simulink model "plant"  (R2026a)
settings: Solver=VariableStepAuto  StopTime=11
InitFcn:
  | run('plant_parameters.m');
values from neighbouring files (symbols this model uses):
  d = 0.1845    [plant_parameters.m]
  dd = d / sqrt(2)    [plant_parameters.m]
  Kd_J1 = 40    [plant_parameters.m]
  Kd_J2 = 30    [plant_parameters.m]
  Kd_J3 = 12    [plant_parameters.m]
  Ki_J1 = 800    [plant_parameters.m]
  Ki_J2 = 700    [plant_parameters.m]
  Ki_J3 = 300    [plant_parameters.m]
  Kp_J1 = 800    [plant_parameters.m]
  Kp_J2 = 600    [plant_parameters.m]
  Kp_J3 = 250    [plant_parameters.m]
  L1 = 0.074    [plant_parameters.m]
  L2 = 0.121    [plant_parameters.m]
  L3 = 0.230    (= 0.23)    [plant_parameters.m]
  N_J1 = 120    [plant_parameters.m]
  N_J2 = 120    [plant_parameters.m]
  N_J3 = 120    [plant_parameters.m]
  Sampling_Time = 0.005    [plant_parameters.m]
undefined symbols (not defined in the file or in its folder): X, Y, Z
libraries: sm_lib x121, nesl_utility x55, slpidlib x18
(part 7 of 8)

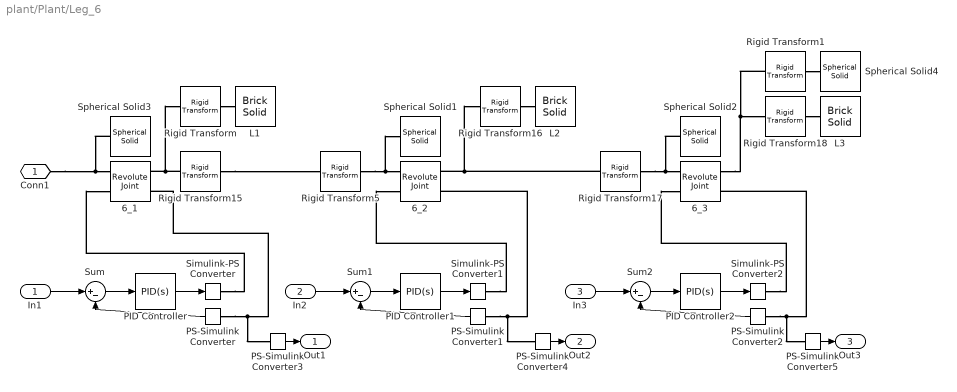
== system plant/Plant/Leg_6 ==
  In1 : Inport
  In2 : Inport  Port=2
  In3 : Inport  Port=3
  6_1 : sm_lib/Joints/Revolute Joint  JointMode=Normal  CompositeWrenchDir=FollowerOnBase  CompositeWrenchFrame=BaseFrame  SenseConstraintForce=off  SenseConstraintTorque=off  SenseTotalForce=off  SenseTotalTorque=off  PositionTargetSpecify=off  PositionTargetPriority=High  PositionTargetValue=0  PositionTargetValueUnits=deg  VelocityTargetSpecify=off  VelocityTargetPriority=High  VelocityTargetValue=0  VelocityTargetValueUnits=deg/s  EquilibriumPosition=0  EquilibriumPositionUnits=deg  SpringStiffness=0  SpringStiffnessUnits=N*m/deg  DampingCoefficient=0  DampingCoefficientUnits=N*m/(deg/s)  LowerLimitSpecify=off  LowerLimitBound=-90  LowerLimitBoundUnits=deg  LowerLimitStiffness=1e4  LowerLimitStiffnessUnits=N*m/deg  LowerLimitDamping=10  LowerLimitDampingUnits=N*m/(deg/s)  LowerLimitTransitionRegionWidth=0.1  LowerLimitTransitionRegionWidthUnits=deg  UpperLimitSpecify=off  UpperLimitBound=90  UpperLimitBoundUnits=deg  UpperLimitStiffness=1e4  UpperLimitStiffnessUnits=N*m/deg  UpperLimitDamping=10  UpperLimitDampingUnits=N*m/(deg/s)  UpperLimitTransitionRegionWidth=0.1  UpperLimitTransitionRegionWidthUnits=deg  TorqueActuationMode=InputTorque  MotionActuationMode=ComputedMotion  SensePosition=on  SenseVelocity=off  SenseAcceleration=off  SenseTorqueForce=off  SenseLowerLimitTorqueForce=off  SenseUpperLimitTorqueForce=off
  6_2 : sm_lib/Joints/Revolute Joint  JointMode=Normal  CompositeWrenchDir=FollowerOnBase  CompositeWrenchFrame=BaseFrame  SenseConstraintForce=off  SenseConstraintTorque=off  SenseTotalForce=off  SenseTotalTorque=off  PositionTargetSpecify=off  PositionTargetPriority=High  PositionTargetValue=0  PositionTargetValueUnits=deg  VelocityTargetSpecify=off  VelocityTargetPriority=High  VelocityTargetValue=0  VelocityTargetValueUnits=deg/s  EquilibriumPosition=0  EquilibriumPositionUnits=deg  SpringStiffness=0  SpringStiffnessUnits=N*m/deg  DampingCoefficient=0  DampingCoefficientUnits=N*m/(deg/s)  LowerLimitSpecify=off  LowerLimitBound=-90  LowerLimitBoundUnits=deg  LowerLimitStiffness=1e4  LowerLimitStiffnessUnits=N*m/deg  LowerLimitDamping=10  LowerLimitDampingUnits=N*m/(deg/s)  LowerLimitTransitionRegionWidth=0.1  LowerLimitTransitionRegionWidthUnits=deg  UpperLimitSpecify=off  UpperLimitBound=90  UpperLimitBoundUnits=deg  UpperLimitStiffness=1e4  UpperLimitStiffnessUnits=N*m/deg  UpperLimitDamping=10  UpperLimitDampingUnits=N*m/(deg/s)  UpperLimitTransitionRegionWidth=0.1  UpperLimitTransitionRegionWidthUnits=deg  TorqueActuationMode=InputTorque  MotionActuationMode=ComputedMotion  SensePosition=on  SenseVelocity=off  SenseAcceleration=off  SenseTorqueForce=off  SenseLowerLimitTorqueForce=off  SenseUpperLimitTorqueForce=off
  6_3 : sm_lib/Joints/Revolute Joint  JointMode=Normal  CompositeWrenchDir=FollowerOnBase  CompositeWrenchFrame=BaseFrame  SenseConstraintForce=off  SenseConstraintTorque=off  SenseTotalForce=off  SenseTotalTorque=off  PositionTargetSpecify=off  PositionTargetPriority=High  PositionTargetValue=0  PositionTargetValueUnits=deg  VelocityTargetSpecify=off  VelocityTargetPriority=High  VelocityTargetValue=0  VelocityTargetValueUnits=deg/s  EquilibriumPosition=0  EquilibriumPositionUnits=deg  SpringStiffness=0  SpringStiffnessUnits=N*m/deg  DampingCoefficient=0  DampingCoefficientUnits=N*m/(deg/s)  LowerLimitSpecify=off  LowerLimitBound=-90  LowerLimitBoundUnits=deg  LowerLimitStiffness=1e4  LowerLimitStiffnessUnits=N*m/deg  LowerLimitDamping=10  LowerLimitDampingUnits=N*m/(deg/s)  LowerLimitTransitionRegionWidth=0.1  LowerLimitTransitionRegionWidthUnits=deg  UpperLimitSpecify=off  UpperLimitBound=90  UpperLimitBoundUnits=deg  UpperLimitStiffness=1e4  UpperLimitStiffnessUnits=N*m/deg  UpperLimitDamping=10  UpperLimitDampingUnits=N*m/(deg/s)  UpperLimitTransitionRegionWidth=0.1  UpperLimitTransitionRegionWidthUnits=deg  TorqueActuationMode=InputTorque  MotionActuationMode=ComputedMotion  SensePosition=on  SenseVelocity=off  SenseAcceleration=off  SenseTorqueForce=off  SenseLowerLimitTorqueForce=off  SenseUpperLimitTorqueForce=off
  L1 : sm_lib/Body Elements/Brick Solid  BrickDimensions=[L1 0.05 0.05]  BrickDimensionsUnits=m  ExportEntireGeometry=off  InertiaType=CalculateFromGeometry  BasedOnType=Density  Density=1000  DensityUnits=kg/m^3  Mass=1  MassUnits=kg  CenterOfMass=[0 0 0]  CenterOfMassUnits=m  MomentsOfInertia=[1 1 1]  MomentsOfInertiaUnits=kg*m^2  ProductsOfInertia=[0 0 0]  ProductsOfInertiaUnits=kg*m^2  GraphicType=FromGeometry  MarkerShape=Sphere  MarkerSize=10  GraphicVisPropType=SimpleVisualProperties  GraphicDiffuseColor=[0.5 0.5 0.5]  GraphicOpacity=1  GraphicSpecularColor=[0.5 0.5 0.5 1.0]  GraphicAmbientColor=[0.15 0.15 0.15 1.0]  GraphicEmissiveColor=[0.0 0.0 0.0 1.0]  GraphicShininess=75  DoExposeReferenceFrame=on  SerializedFrames=<Frames/>
  L2 : sm_lib/Body Elements/Brick Solid  BrickDimensions=[L2 0.05 0.05]  BrickDimensionsUnits=m  ExportEntireGeometry=off  InertiaType=CalculateFromGeometry  BasedOnType=Density  Density=1000  DensityUnits=kg/m^3  Mass=1  MassUnits=kg  CenterOfMass=[0 0 0]  CenterOfMassUnits=m  MomentsOfInertia=[1 1 1]  MomentsOfInertiaUnits=kg*m^2  ProductsOfInertia=[0 0 0]  ProductsOfInertiaUnits=kg*m^2  GraphicType=FromGeometry  MarkerShape=Sphere  MarkerSize=10  GraphicVisPropType=SimpleVisualProperties  GraphicDiffuseColor=[0.5 0.5 0.5]  GraphicOpacity=1  GraphicSpecularColor=[0.5 0.5 0.5 1.0]  GraphicAmbientColor=[0.15 0.15 0.15 1.0]  GraphicEmissiveColor=[0.0 0.0 0.0 1.0]  GraphicShininess=75  DoExposeReferenceFrame=on  SerializedFrames=<Frames/>
  L3 : sm_lib/Body Elements/Brick Solid  BrickDimensions=[L3 0.05 0.05]  BrickDimensionsUnits=m  ExportEntireGeometry=off  InertiaType=CalculateFromGeometry  BasedOnType=Density  Density=1000  DensityUnits=kg/m^3  Mass=1  MassUnits=kg  CenterOfMass=[0 0 0]  CenterOfMassUnits=m  MomentsOfInertia=[1 1 1]  MomentsOfInertiaUnits=kg*m^2  ProductsOfInertia=[0 0 0]  ProductsOfInertiaUnits=kg*m^2  GraphicType=FromGeometry  MarkerShape=Sphere  MarkerSize=10  GraphicVisPropType=SimpleVisualProperties  GraphicDiffuseColor=[0.5 0.5 0.5]  GraphicOpacity=1  GraphicSpecularColor=[0.5 0.5 0.5 1.0]  GraphicAmbientColor=[0.15 0.15 0.15 1.0]  GraphicEmissiveColor=[0.0 0.0 0.0 1.0]  GraphicShininess=75  DoExposeReferenceFrame=on  SerializedFrames=<Frames/>
  PID Controller : slpidlib/PID Controller  Controller=PID  Form=Parallel  TimeDomain=Continuous-time  UseExternalTs=off  SampleTime=-1  IntegratorMethod=Forward Euler  FilterMethod=Forward Euler  ControllerParametersSource=internal  P=Kp_J1  I=Ki_J1  UseKiTs=off  D=Kd_J1  UseExternalDerivativeSource=off  N=N_J1  UseFilter=on  TunerSelectOption=Transfer Function Based (PID Tuner App)  InitialConditionSource=internal  InitialConditionForIntegrator=0  InitialConditionForFilter=0  DifferentiatorICPrevScaledInput=0  ExternalReset=none  TrackingMode=off  Kt=1  LimitOutput=off  SatLimitsSource=internal  UpperSaturationLimit=inf  LowerSaturationLimit=-inf  LinearizeAsGain=on  AntiWindupMode=none  Kb=1  LimitIntegrator=off  UpperIntegratorSaturationLimit=inf  LowerIntegratorSaturationLimit=-inf  POutMin=[]  POutMax=[]  IOutMin=[]  IOutMax=[]  DOutMin=[]  DOutMax=[]  NOutMin=[]  NOutMax=[]  SumOutMin=[]  SumOutMax=[]  SaturationOutMin=[]  SaturationOutMax=[]  PParamMin=[]  PParamMax=[]  IParamMin=[]  IParamMax=[]  DParamMin=[]  DParamMax=[]  NParamMin=[]  NParamMax=[]  KbParamMin=[]  KbParamMax=[]  KtParamMin=[]  KtParamMax=[]  KbOutMin=[]  KbOutMax=[]  KtOutMin=[]  KtOutMax=[]  IntegratorOutMin=[]  IntegratorOutMax=[]  FilterOutMin=[]  FilterOutMax=[]  SumI1OutMin=[]  SumI1OutMax=[]  SumI2OutMin=[]  SumI2OutMax=[]  SumI3OutMin=[]  SumI3OutMax=[]  SumI4OutMin=[]  SumI4OutMax=[]  SumDOutMin=[]  SumDOutMax=[]  DifferentiatorOutMin=[]  DifferentiatorOutMax=[]  FilterDiffOutCoefMin=[]  FilterDiffOutCoefMax=[]  ReciprocalOutMin=[]  ReciprocalOutMax=[]  SumDenOutMin=[]  SumDenOutMax=[]  SumNumOutMin=[]  SumNumOutMax=[]  DivideOutMin=[]  DivideOutMax=[]  UdiffTsProdOutMin=[]  UdiffTsProdOutMax=[]  NTsProdOutMin=[]  NTsProdOutMax=[]  UintegralTsProdOutMin=[]  UintegralTsProdOutMax=[]  UngainTsProdOutMin=[]  UngainTsProdOutMax=[]  ClampingZeroOutDataTypeStr=Inherit: Inherit via back propagation  ClampingZeroOutMin=[]  ClampingZeroOutMax=[]  FilterDenConstantOutDataTypeStr=Inherit: Inherit via back propagation  FilterDenConstantOutMin=[]  FilterDenConstantOutMax=[]  PCopyOutDataTypeStr=Inherit: Inherit via back propagation  PCopyOutMin=[]  PCopyOutMax=[]  NCopyOutDataTypeStr=Inherit: Inherit via back propagation  NCopyOutMin=[]  NCopyOutMax=[]  IntegratorContinuousStateAttributes=''  IntegratorStateMustResolveToSignalObject=off  IntegratorRTWStateStorageClass=Auto  FilterContinuousStateAttributes=''  FilterStateMustResolveToSignalObject=off  FilterRTWStateStorageClass=Auto  ParallelPVariant=InternalParameters  IdealPVariant=Disabled  IVariant=InternalParameters  DVariant=InternalParameters  IntegratorVariant=Continuous  SatVariant=Disabled  AWVariant=Passthrough  PCopyVariant=Disabled  TRVariant=Disabled  FdbkBlocksVariant=Forward  IdealPFdbkVariant=Disabled  SatFdbkVariant=Disabled  DerivativeFilterVariant=ContFilter  NVariant=InternalParameters  NCopyVariant=Disabled  FilterICVariant=InternalICsFilter  IntegratorICVariant=InternalICs  ExternalResetVariant=Disabled  TRSumVariant=Passthrough  SumFdbkVariant=Disabled  SumVariant=Sum_PID  TsampFilterVariant=InternalTs  TsampNgainVariant=Passthrough  TsampIntegralVariant=Disabled_SignalSpec  ExternalSaturationOutDataTypeStr=Inherit: Same as second input  DerivativeSourceVariant=ErrorSignal  PreIntVariant=InternalPreInt
  PID Controller1 : slpidlib/PID Controller  Controller=PID  Form=Parallel  TimeDomain=Continuous-time  UseExternalTs=off  SampleTime=-1  IntegratorMethod=Forward Euler  FilterMethod=Forward Euler  ControllerParametersSource=internal  P=Kp_J2  I=Ki_J2  UseKiTs=off  D=Kd_J2  UseExternalDerivativeSource=off  N=N_J2  UseFilter=on  TunerSelectOption=Transfer Function Based (PID Tuner App)  InitialConditionSource=internal  InitialConditionForIntegrator=0  InitialConditionForFilter=0  DifferentiatorICPrevScaledInput=0  ExternalReset=none  TrackingMode=off  Kt=1  LimitOutput=off  SatLimitsSource=internal  UpperSaturationLimit=inf  LowerSaturationLimit=-inf  LinearizeAsGain=on  AntiWindupMode=none  Kb=1  LimitIntegrator=off  UpperIntegratorSaturationLimit=inf  LowerIntegratorSaturationLimit=-inf  POutMin=[]  POutMax=[]  IOutMin=[]  IOutMax=[]  DOutMin=[]  DOutMax=[]  NOutMin=[]  NOutMax=[]  SumOutMin=[]  SumOutMax=[]  SaturationOutMin=[]  SaturationOutMax=[]  PParamMin=[]  PParamMax=[]  IParamMin=[]  IParamMax=[]  DParamMin=[]  DParamMax=[]  NParamMin=[]  NParamMax=[]  KbParamMin=[]  KbParamMax=[]  KtParamMin=[]  KtParamMax=[]  KbOutMin=[]  KbOutMax=[]  KtOutMin=[]  KtOutMax=[]  IntegratorOutMin=[]  IntegratorOutMax=[]  FilterOutMin=[]  FilterOutMax=[]  SumI1OutMin=[]  SumI1OutMax=[]  SumI2OutMin=[]  SumI2OutMax=[]  SumI3OutMin=[]  SumI3OutMax=[]  SumI4OutMin=[]  SumI4OutMax=[]  SumDOutMin=[]  SumDOutMax=[]  DifferentiatorOutMin=[]  DifferentiatorOutMax=[]  FilterDiffOutCoefMin=[]  FilterDiffOutCoefMax=[]  ReciprocalOutMin=[]  ReciprocalOutMax=[]  SumDenOutMin=[]  SumDenOutMax=[]  SumNumOutMin=[]  SumNumOutMax=[]  DivideOutMin=[]  DivideOutMax=[]  UdiffTsProdOutMin=[]  UdiffTsProdOutMax=[]  NTsProdOutMin=[]  NTsProdOutMax=[]  UintegralTsProdOutMin=[]  UintegralTsProdOutMax=[]  UngainTsProdOutMin=[]  UngainTsProdOutMax=[]  ClampingZeroOutDataTypeStr=Inherit: Inherit via back propagation  ClampingZeroOutMin=[]  ClampingZeroOutMax=[]  FilterDenConstantOutDataTypeStr=Inherit: Inherit via back propagation  FilterDenConstantOutMin=[]  FilterDenConstantOutMax=[]  PCopyOutDataTypeStr=Inherit: Inherit via back propagation  PCopyOutMin=[]  PCopyOutMax=[]  NCopyOutDataTypeStr=Inherit: Inherit via back propagation  NCopyOutMin=[]  NCopyOutMax=[]  IntegratorContinuousStateAttributes=''  IntegratorStateMustResolveToSignalObject=off  IntegratorRTWStateStorageClass=Auto  FilterContinuousStateAttributes=''  FilterStateMustResolveToSignalObject=off  FilterRTWStateStorageClass=Auto  ParallelPVariant=InternalParameters  IdealPVariant=Disabled  IVariant=InternalParameters  DVariant=InternalParameters  IntegratorVariant=Continuous  SatVariant=Disabled  AWVariant=Passthrough  PCopyVariant=Disabled  TRVariant=Disabled  FdbkBlocksVariant=Forward  IdealPFdbkVariant=Disabled  SatFdbkVariant=Disabled  DerivativeFilterVariant=ContFilter  NVariant=InternalParameters  NCopyVariant=Disabled  FilterICVariant=InternalICsFilter  IntegratorICVariant=InternalICs  ExternalResetVariant=Disabled  TRSumVariant=Passthrough  SumFdbkVariant=Disabled  SumVariant=Sum_PID  TsampFilterVariant=InternalTs  TsampNgainVariant=Passthrough  TsampIntegralVariant=Disabled_SignalSpec  ExternalSaturationOutDataTypeStr=Inherit: Same as second input  DerivativeSourceVariant=ErrorSignal  PreIntVariant=InternalPreInt
  PID Controller2 : slpidlib/PID Controller  Controller=PID  Form=Parallel  TimeDomain=Continuous-time  UseExternalTs=off  SampleTime=-1  IntegratorMethod=Forward Euler  FilterMethod=Forward Euler  ControllerParametersSource=internal  P=Kp_J3  I=Ki_J3  UseKiTs=off  D=Kd_J3  UseExternalDerivativeSource=off  N=N_J3  UseFilter=on  TunerSelectOption=Transfer Function Based (PID Tuner App)  InitialConditionSource=internal  InitialConditionForIntegrator=0  InitialConditionForFilter=0  DifferentiatorICPrevScaledInput=0  ExternalReset=none  TrackingMode=off  Kt=1  LimitOutput=off  SatLimitsSource=internal  UpperSaturationLimit=inf  LowerSaturationLimit=-inf  LinearizeAsGain=on  AntiWindupMode=none  Kb=1  LimitIntegrator=off  UpperIntegratorSaturationLimit=inf  LowerIntegratorSaturationLimit=-inf  POutMin=[]  POutMax=[]  IOutMin=[]  IOutMax=[]  DOutMin=[]  DOutMax=[]  NOutMin=[]  NOutMax=[]  SumOutMin=[]  SumOutMax=[]  SaturationOutMin=[]  SaturationOutMax=[]  PParamMin=[]  PParamMax=[]  IParamMin=[]  IParamMax=[]  DParamMin=[]  DParamMax=[]  NParamMin=[]  NParamMax=[]  KbParamMin=[]  KbParamMax=[]  KtParamMin=[]  KtParamMax=[]  KbOutMin=[]  KbOutMax=[]  KtOutMin=[]  KtOutMax=[]  IntegratorOutMin=[]  IntegratorOutMax=[]  FilterOutMin=[]  FilterOutMax=[]  SumI1OutMin=[]  SumI1OutMax=[]  SumI2OutMin=[]  SumI2OutMax=[]  SumI3OutMin=[]  SumI3OutMax=[]  SumI4OutMin=[]  SumI4OutMax=[]  SumDOutMin=[]  SumDOutMax=[]  DifferentiatorOutMin=[]  DifferentiatorOutMax=[]  FilterDiffOutCoefMin=[]  FilterDiffOutCoefMax=[]  ReciprocalOutMin=[]  ReciprocalOutMax=[]  SumDenOutMin=[]  SumDenOutMax=[]  SumNumOutMin=[]  SumNumOutMax=[]  DivideOutMin=[]  DivideOutMax=[]  UdiffTsProdOutMin=[]  UdiffTsProdOutMax=[]  NTsProdOutMin=[]  NTsProdOutMax=[]  UintegralTsProdOutMin=[]  UintegralTsProdOutMax=[]  UngainTsProdOutMin=[]  UngainTsProdOutMax=[]  ClampingZeroOutDataTypeStr=Inherit: Inherit via back propagation  ClampingZeroOutMin=[]  ClampingZeroOutMax=[]  FilterDenConstantOutDataTypeStr=Inherit: Inherit via back propagation  FilterDenConstantOutMin=[]  FilterDenConstantOutMax=[]  PCopyOutDataTypeStr=Inherit: Inherit via back propagation  PCopyOutMin=[]  PCopyOutMax=[]  NCopyOutDataTypeStr=Inherit: Inherit via back propagation  NCopyOutMin=[]  NCopyOutMax=[]  IntegratorContinuousStateAttributes=''  IntegratorStateMustResolveToSignalObject=off  IntegratorRTWStateStorageClass=Auto  FilterContinuousStateAttributes=''  FilterStateMustResolveToSignalObject=off  FilterRTWStateStorageClass=Auto  ParallelPVariant=InternalParameters  IdealPVariant=Disabled  IVariant=InternalParameters  DVariant=InternalParameters  IntegratorVariant=Continuous  SatVariant=Disabled  AWVariant=Passthrough  PCopyVariant=Disabled  TRVariant=Disabled  FdbkBlocksVariant=Forward  IdealPFdbkVariant=Disabled  SatFdbkVariant=Disabled  DerivativeFilterVariant=ContFilter  NVariant=InternalParameters  NCopyVariant=Disabled  FilterICVariant=InternalICsFilter  IntegratorICVariant=InternalICs  ExternalResetVariant=Disabled  TRSumVariant=Passthrough  SumFdbkVariant=Disabled  SumVariant=Sum_PID  TsampFilterVariant=InternalTs  TsampNgainVariant=Passthrough  TsampIntegralVariant=Disabled_SignalSpec  ExternalSaturationOutDataTypeStr=Inherit: Same as second input  DerivativeSourceVariant=ErrorSignal  PreIntVariant=InternalPreInt
  PS-Simulink Converter{,1..5} (6 alike) : nesl_utility/PS-Simulink Converter  PhysicalDomain=network_engine_domain  SubClassName=ps_output  LeftPortType=input  RightPortType=output  PseudoPeriodic=off  Frequencies=[]  VectorFormat=inherit  Unit=inherit  AffineConversion=off
  Rigid Transform : sm_lib/Frames and Transforms/Rigid Transform  RotationMethod=None  FollAlignAxisA=+X  BaseAlignAxisA=+Y  FollAlignAxisB=+Y  BaseAlignAxisB=+Z  RotationStandardAxis=+Z  RotationAngle=0  RotationAngleUnits=deg  RotationArbitraryAxis=[0 0 1]  RotationSequenceAxes=FollowerAxes  RotationSequence=XYX  RotationSequenceAngles=[0 0 0]  RotationSequenceAnglesUnits=deg  RotationMatrix=[1 0 0;0 1 0;0 0 1]  Quaternion=[1 0 0 0]  TranslationMethod=Cartesian  TranslationCartesianOffset=[L1/2 0 0]  TranslationCartesianOffsetUnits=m  TranslationStandardAxis=+Z  TranslationStandardOffset=0  TranslationStandardOffsetUnits=m  TranslationROffset=0  TranslationROffsetUnits=m  TranslationThetaOffset=0  TranslationThetaOffsetUnits=deg  TranslationZOffset=0  TranslationZOffsetUnits=m
  Rigid Transform1 : sm_lib/Frames and Transforms/Rigid Transform  RotationMethod=None  FollAlignAxisA=+X  BaseAlignAxisA=+Y  FollAlignAxisB=+Y  BaseAlignAxisB=+Z  RotationStandardAxis=+Z  RotationAngle=0  RotationAngleUnits=deg  RotationArbitraryAxis=[0 0 1]  RotationSequenceAxes=FollowerAxes  RotationSequence=XYX  RotationSequenceAngles=[0 0 0]  RotationSequenceAnglesUnits=deg  RotationMatrix=[1 0 0;0 1 0;0 0 1]  Quaternion=[1 0 0 0]  TranslationMethod=Cartesian  TranslationCartesianOffset=[L3 0 0]  TranslationCartesianOffsetUnits=m  TranslationStandardAxis=+Z  TranslationStandardOffset=0  TranslationStandardOffsetUnits=m  TranslationROffset=0  TranslationROffsetUnits=m  TranslationThetaOffset=0  TranslationThetaOffsetUnits=deg  TranslationZOffset=0  TranslationZOffsetUnits=m
  Rigid Transform15 : sm_lib/Frames and Transforms/Rigid Transform  RotationMethod=None  FollAlignAxisA=+X  BaseAlignAxisA=+Y  FollAlignAxisB=+Y  BaseAlignAxisB=+Z  RotationStandardAxis=+Z  RotationAngle=0  RotationAngleUnits=deg  RotationArbitraryAxis=[0 0 1]  RotationSequenceAxes=FollowerAxes  RotationSequence=XYX  RotationSequenceAngles=[0 0 0]  RotationSequenceAnglesUnits=deg  RotationMatrix=[1 0 0;0 1 0;0 0 1]  Quaternion=[1 0 0 0]  TranslationMethod=Cartesian  TranslationCartesianOffset=[L1 0 0]  TranslationCartesianOffsetUnits=m  TranslationStandardAxis=+Z  TranslationStandardOffset=0  TranslationStandardOffsetUnits=m  TranslationROffset=0  TranslationROffsetUnits=m  TranslationThetaOffset=0  TranslationThetaOffsetUnits=deg  TranslationZOffset=0  TranslationZOffsetUnits=m
  Rigid Transform16 : sm_lib/Frames and Transforms/Rigid Transform  RotationMethod=None  FollAlignAxisA=+X  BaseAlignAxisA=+Y  FollAlignAxisB=+Y  BaseAlignAxisB=+Z  RotationStandardAxis=+Z  RotationAngle=0  RotationAngleUnits=deg  RotationArbitraryAxis=[0 0 1]  RotationSequenceAxes=FollowerAxes  RotationSequence=XYX  RotationSequenceAngles=[0 0 0]  RotationSequenceAnglesUnits=deg  RotationMatrix=[1 0 0;0 1 0;0 0 1]  Quaternion=[1 0 0 0]  TranslationMethod=Cartesian  TranslationCartesianOffset=[L2/2 0 0]  TranslationCartesianOffsetUnits=m  TranslationStandardAxis=+Z  TranslationStandardOffset=0  TranslationStandardOffsetUnits=m  TranslationROffset=0  TranslationROffsetUnits=m  TranslationThetaOffset=0  TranslationThetaOffsetUnits=deg  TranslationZOffset=0  TranslationZOffsetUnits=m
  Rigid Transform17 : sm_lib/Frames and Transforms/Rigid Transform  RotationMethod=None  FollAlignAxisA=+X  BaseAlignAxisA=+Y  FollAlignAxisB=+Y  BaseAlignAxisB=+Z  RotationStandardAxis=+Z  RotationAngle=0  RotationAngleUnits=deg  RotationArbitraryAxis=[0 0 1]  RotationSequenceAxes=FollowerAxes  RotationSequence=XYX  RotationSequenceAngles=[0 0 0]  RotationSequenceAnglesUnits=deg  RotationMatrix=[1 0 0;0 1 0;0 0 1]  Quaternion=[1 0 0 0]  TranslationMethod=Cartesian  TranslationCartesianOffset=[L2 0 0]  TranslationCartesianOffsetUnits=m  TranslationStandardAxis=+Z  TranslationStandardOffset=0  TranslationStandardOffsetUnits=m  TranslationROffset=0  TranslationROffsetUnits=m  TranslationThetaOffset=0  TranslationThetaOffsetUnits=deg  TranslationZOffset=0  TranslationZOffsetUnits=m
  Rigid Transform18 : sm_lib/Frames and Transforms/Rigid Transform  RotationMethod=None  FollAlignAxisA=+X  BaseAlignAxisA=+Y  FollAlignAxisB=+Y  BaseAlignAxisB=+Z  RotationStandardAxis=+Z  RotationAngle=0  RotationAngleUnits=deg  RotationArbitraryAxis=[0 0 1]  RotationSequenceAxes=FollowerAxes  RotationSequence=XYX  RotationSequenceAngles=[0 0 0]  RotationSequenceAnglesUnits=deg  RotationMatrix=[1 0 0;0 1 0;0 0 1]  Quaternion=[1 0 0 0]  TranslationMethod=Cartesian  TranslationCartesianOffset=[L3/2 0 0]  TranslationCartesianOffsetUnits=m  TranslationStandardAxis=+Z  TranslationStandardOffset=0  TranslationStandardOffsetUnits=m  TranslationROffset=0  TranslationROffsetUnits=m  TranslationThetaOffset=0  TranslationThetaOffsetUnits=deg  TranslationZOffset=0  TranslationZOffsetUnits=m
  Rigid Transform5 : sm_lib/Frames and Transforms/Rigid Transform  RotationMethod=StandardAxis  FollAlignAxisA=+X  BaseAlignAxisA=+Y  FollAlignAxisB=+Y  BaseAlignAxisB=+Z  RotationStandardAxis=-X  RotationAngle=90  RotationAngleUnits=deg  RotationArbitraryAxis=[0 0 1]  RotationSequenceAxes=FollowerAxes  RotationSequence=XYX  RotationSequenceAngles=[0 0 0]  RotationSequenceAnglesUnits=deg  RotationMatrix=[1 0 0;0 1 0;0 0 1]  Quaternion=[1 0 0 0]  TranslationMethod=None  TranslationCartesianOffset=[L1 0 0]  TranslationCartesianOffsetUnits=m  TranslationStandardAxis=+Z  TranslationStandardOffset=0  TranslationStandardOffsetUnits=m  TranslationROffset=0  TranslationROffsetUnits=m  TranslationThetaOffset=0  TranslationThetaOffsetUnits=deg  TranslationZOffset=0  TranslationZOffsetUnits=m
  Simulink-PS Converter : nesl_utility/Simulink-PS Converter  PhysicalDomain=network_engine_domain  SubClassName=ps_input  LeftPortType=input  RightPortType=output  PseudoPeriodic=off  Frequencies=[]  NoiseDistribution=none  NoiseParameters=[]  Unit=1  AffineConversion=off  FilteringAndDerivatives=provide  SimscapeFilterOrder=1  InputFilterTimeConstant=0.001  UdotUserProvided=0
  Simulink-PS Converter1 : nesl_utility/Simulink-PS Converter  PhysicalDomain=network_engine_domain  SubClassName=ps_input  LeftPortType=input  RightPortType=output  PseudoPeriodic=off  Frequencies=[]  NoiseDistribution=none  NoiseParameters=[]  Unit=1  AffineConversion=off  FilteringAndDerivatives=provide  SimscapeFilterOrder=1  InputFilterTimeConstant=0.001  UdotUserProvided=0
  Simulink-PS Converter2 : nesl_utility/Simulink-PS Converter  PhysicalDomain=network_engine_domain  SubClassName=ps_input  LeftPortType=input  RightPortType=output  PseudoPeriodic=off  Frequencies=[]  NoiseDistribution=none  NoiseParameters=[]  Unit=1  AffineConversion=off  FilteringAndDerivatives=provide  SimscapeFilterOrder=1  InputFilterTimeConstant=0.001  UdotUserProvided=0
  Spherical Solid{1..4} (4 alike) : sm_lib/Body Elements/Spherical Solid  SphereRadius=0.044  SphereRadiusUnits=m  ExportEntireGeometry=off  InertiaType=CalculateFromGeometry  BasedOnType=Density  Density=1000  DensityUnits=kg/m^3  Mass=1  MassUnits=kg  CenterOfMass=[0 0 0]  CenterOfMassUnits=m  MomentsOfInertia=[1 1 1]  MomentsOfInertiaUnits=kg*m^2  ProductsOfInertia=[0 0 0]  ProductsOfInertiaUnits=kg*m^2  GraphicType=FromGeometry  MarkerShape=Sphere  MarkerSize=10  GraphicVisPropType=SimpleVisualProperties  GraphicDiffuseColor=[0 0.3333 1]  GraphicOpacity=1  GraphicSpecularColor=[0.5 0.5 0.5 1.0]  GraphicAmbientColor=[0.15 0.15 0.15 1.0]  GraphicEmissiveColor=[0.0 0.0 0.0 1.0]  GraphicShininess=75  DoExposeReferenceFrame=on  SerializedFrames=<Frames/>
  Sum : Sum  Inputs=|+-
  Sum1 : Sum  Inputs=|+-
  Sum2 : Sum  Inputs=|+-
  Conn1 : PMIOPort  Side=Left
  Out1 : Outport
  Out2 : Outport  Port=2
  Out3 : Outport  Port=3
  wires:
  PID Controller/1 -> Simulink-PS Converter/1
  Sum1/1 -> PID Controller1/1
  In2/1 -> Sum1/1
  Sum/1 -> PID Controller/1
  In3/1 -> Sum2/1
  PID Controller2/1 -> Simulink-PS Converter2/1
  In1/1 -> Sum/1
  PS-Simulink Converter/1 -> Sum/2
  PS-Simulink Converter1/1 -> Sum1/2
  PS-Simulink Converter2/1 -> Sum2/2
  Sum2/1 -> PID Controller2/1
  PID Controller1/1 -> Simulink-PS Converter1/1
  PS-Simulink Converter3/1 -> Out1/1
  PS-Simulink Converter4/1 -> Out2/1
  PS-Simulink Converter5/1 -> Out3/1
  connections:
  Rigid Transform/RConn1 -- L1/RConn1
  Rigid Transform16/RConn1 -- L2/RConn1
  Rigid Transform15/RConn1 -- Rigid Transform5/LConn1
  6_3/RConn2 -- PS-Simulink Converter2/LConn1 -- PS-Simulink Converter5/LConn1
  Rigid Transform17/LConn1 -- Rigid Transform16/LConn1 -- 6_2/RConn1
  Rigid Transform17/RConn1 -- Spherical Solid2/RConn1 -- 6_3/LConn1
  Rigid Transform5/RConn1 -- Spherical Solid1/RConn1 -- 6_2/LConn1
  Simulink-PS Converter/RConn1 -- 6_1/LConn2
  Simulink-PS Converter1/RConn1 -- 6_2/LConn2
  6_3/RConn1 -- Rigid Transform1/LConn1 -- Rigid Transform18/LConn1
  Rigid Transform15/LConn1 -- Rigid Transform/LConn1 -- 6_1/RConn1
  Rigid Transform18/RConn1 -- L3/RConn1
  6_2/RConn2 -- PS-Simulink Converter1/LConn1 -- PS-Simulink Converter4/LConn1
  PS-Simulink Converter/LConn1 -- 6_1/RConn2 -- PS-Simulink Converter3/LConn1
  Conn1/RConn1 -- Spherical Solid3/RConn1 -- 6_1/LConn1
  Simulink-PS Converter2/RConn1 -- 6_3/LConn2
  Rigid Transform1/RConn1 -- Spherical Solid4/RConn1

== matlab function plant/MATLAB Function2 ==
  data: xL output; yL output; q1 input; q2 input; q3 input; zL output
function [xL, yL, zL] = legFK(q1, q2, q3)
% 현재 관절각으로 발끝 위치를 계산한다.

L1 = 0.074;   % 링크1 에서 링크1 까지 거리 (m)
L2 = 0.121;   % 링크2 에서 링크3 까지 거리 (m)
L3 = 0.230;   % 링크3 에서 발 끝 까지 거리 (m)

r = L1 + L2*cos(q2) + L3*cos(q2 + q3);    % 수평 도달 거리를 계산한다.

xL = r*cos(q1);                            % 다리 좌표계 x 위치를 계산한다.
yL = r*sin(q1);                            % 다리 좌표계 y 위치를 계산한다.
zL = -L2*sin(q2) - L3*sin(q2 + q3);        % 다리 좌표계 z 위치를 계산한다.
end

== matlab function plant/MATLAB Function3 ==
  data: xL output; yL output; q1 input; q2 input; q3 input; zL output
function [xL, yL, zL] = legFK(q1, q2, q3)
% 현재 관절각으로 발끝 위치를 계산한다.

L1 = 0.074;   % 링크1 에서 링크1 까지 거리 (m)
L2 = 0.121;   % 링크2 에서 링크3 까지 거리 (m)
L3 = 0.230;   % 링크3 에서 발 끝 까지 거리 (m)

r = L1 + L2*cos(q2) + L3*cos(q2 + q3);    % 수평 도달 거리를 계산한다.

xL = r*cos(q1);                            % 다리 좌표계 x 위치를 계산한다.
yL = r*sin(q1);                            % 다리 좌표계 y 위치를 계산한다.
zL = -L2*sin(q2) - L3*sin(q2 + q3);        % 다리 좌표계 z 위치를 계산한다.
end

== matlab function plant/MATLAB Function4 ==
  data: xL output; yL output; q1 input; q2 input; q3 input; zL output
function [xL, yL, zL] = legFK(q1, q2, q3)
% 현재 관절각으로 발끝 위치를 계산한다.

L1 = 0.074;   % 링크1 에서 링크1 까지 거리 (m)
L2 = 0.121;   % 링크2 에서 링크3 까지 거리 (m)
L3 = 0.230;   % 링크3 에서 발 끝 까지 거리 (m)

r = L1 + L2*cos(q2) + L3*cos(q2 + q3);    % 수평 도달 거리를 계산한다.

xL = r*cos(q1);                            % 다리 좌표계 x 위치를 계산한다.
yL = r*sin(q1);                            % 다리 좌표계 y 위치를 계산한다.
zL = -L2*sin(q2) - L3*sin(q2 + q3);        % 다리 좌표계 z 위치를 계산한다.
end

== matlab function plant/MATLAB Function5 ==
  data: xL output; yL output; q1 input; q2 input; q3 input; zL output
function [xL, yL, zL] = legFK(q1, q2, q3)
% 현재 관절각으로 발끝 위치를 계산한다.

L1 = 0.074;   % 링크1 에서 링크1 까지 거리 (m)
L2 = 0.121;   % 링크2 에서 링크3 까지 거리 (m)
L3 = 0.230;   % 링크3 에서 발 끝 까지 거리 (m)

r = L1 + L2*cos(q2) + L3*cos(q2 + q3);    % 수평 도달 거리를 계산한다.

xL = r*cos(q1);                            % 다리 좌표계 x 위치를 계산한다.
yL = r*sin(q1);                            % 다리 좌표계 y 위치를 계산한다.
zL = -L2*sin(q2) - L3*sin(q2 + q3);        % 다리 좌표계 z 위치를 계산한다.
end

== matlab function plant/MATLAB Function6 ==
  data: xL output; yL output; q1 input; q2 input; q3 input; zL output
function [xL, yL, zL] = legFK(q1, q2, q3)
% 현재 관절각으로 발끝 위치를 계산한다.

L1 = 0.074;   % 링크1 에서 링크1 까지 거리 (m)
L2 = 0.121;   % 링크2 에서 링크3 까지 거리 (m)
L3 = 0.230;   % 링크3 에서 발 끝 까지 거리 (m)

r = L1 + L2*cos(q2) + L3*cos(q2 + q3);    % 수평 도달 거리를 계산한다.

xL = r*cos(q1);                            % 다리 좌표계 x 위치를 계산한다.
yL = r*sin(q1);                            % 다리 좌표계 y 위치를 계산한다.
zL = -L2*sin(q2) - L3*sin(q2 + q3);        % 다리 좌표계 z 위치를 계산한다.
end

== matlab function plant/MATLAB Function7 ==
  data: xL input; xB output; yL input; zL input; yB output; zB output
function [xB, yB, zB] = legToBody(xL, yL, zL)
% 다리 좌표의 발 위치를 Body 좌표로 변환한다.

% 몸체의 원점에서 링크1 까지 거리 (m)
d = 0.1845;
dd = d / sqrt(2);

ox = dd;
oy = -dd;
alpha = -pi/4;

xB = ox + xL*cos(alpha) - yL*sin(alpha);    % Body x 위치를 계산한다.
yB = oy + xL*sin(alpha) + yL*cos(alpha);    % Body y 위치를 계산한다.
zB = zL;                                    % Body z 위치를 전달한다.
end

== matlab function plant/MATLAB Function8 ==
  data: xL input; xB output; yL input; zL input; yB output; zB output
function [xB, yB, zB] = legToBody(xL, yL, zL)
% 다리 좌표의 발 위치를 Body 좌표로 변환한다.

% 몸체의 원점에서 링크1 까지 거리 (m)
d = 0.1845;
dd = d / sqrt(2);

ox = 0;
oy = -d;
alpha = -pi/2;

xB = ox + xL*cos(alpha) - yL*sin(alpha);    % Body x 위치를 계산한다.
yB = oy + xL*sin(alpha) + yL*cos(alpha);    % Body y 위치를 계산한다.
zB = zL;                                    % Body z 위치를 전달한다.
end

== matlab function plant/MATLAB Function9 ==
  data: xL input; xB output; yL input; zL input; yB output; zB output
function [xB, yB, zB] = legToBody(xL, yL, zL)
% 다리 좌표의 발 위치를 Body 좌표로 변환한다.

% 몸체의 원점에서 링크1 까지 거리 (m)
d = 0.1845;
dd = d / sqrt(2);

ox = -dd;
oy = -dd;
alpha = -3*pi/4;

xB = ox + xL*cos(alpha) - yL*sin(alpha);    % Body x 위치를 계산한다.
yB = oy + xL*sin(alpha) + yL*cos(alpha);    % Body y 위치를 계산한다.
zB = zL;                                    % Body z 위치를 전달한다.
end

== matlab function plant/MATLAB Function10 ==
  data: xL input; xB output; yL input; zL input; yB output; zB output
function [xB, yB, zB] = legToBody(xL, yL, zL)
% 다리 좌표의 발 위치를 Body 좌표로 변환한다.

% 몸체의 원점에서 링크1 까지 거리 (m)
d = 0.1845;
dd = d / sqrt(2);

ox = dd;
oy = dd;
alpha = pi/4;

xB = ox + xL*cos(alpha) - yL*sin(alpha);    % Body x 위치를 계산한다.
yB = oy + xL*sin(alpha) + yL*cos(alpha);    % Body y 위치를 계산한다.
zB = zL;                                    % Body z 위치를 전달한다.
end

== matlab function plant/MATLAB Function11 ==
  data: xL input; xB output; yL input; zL input; yB output; zB output
function [xB, yB, zB] = legToBody(xL, yL, zL)
% 다리 좌표의 발 위치를 Body 좌표로 변환한다.

% 몸체의 원점에서 링크1 까지 거리 (m)
d = 0.1845;
dd = d / sqrt(2);

ox = 0;
oy = d;
alpha = pi/2;

xB = ox + xL*cos(alpha) - yL*sin(alpha);    % Body x 위치를 계산한다.
yB = oy + xL*sin(alpha) + yL*cos(alpha);    % Body y 위치를 계산한다.
zB = zL;                                    % Body z 위치를 전달한다.
end

== matlab function plant/MATLAB Function12 ==
  data: xL input; xB output; yL input; zL input; yB output; zB output
function [xB, yB, zB] = legToBody(xL, yL, zL)
% 다리 좌표의 발 위치를 Body 좌표로 변환한다.

% 몸체의 원점에서 링크1 까지 거리 (m)
d = 0.1845;
dd = d / sqrt(2);

ox = -dd;
oy = dd;
alpha = 3*pi/4;

xB = ox + xL*cos(alpha) - yL*sin(alpha);    % Body x 위치를 계산한다.
yB = oy + xL*sin(alpha) + yL*cos(alpha);    % Body y 위치를 계산한다.
zB = zL;                                    % Body z 위치를 전달한다.
end

== matlab function plant/MATLAB Function13 ==
  data: xB input; xL output; yB input; zB input; yL output; zL output
function [xL, yL, zL] = bodyToLeg(xB, yB, zB)
% Body 좌표의 발 목표를 다리 좌표로 변환한다.

% 몸체의 원점에서 링크1 까지 거리 (m)
d = 0.1845;
dd = d / sqrt(2);

ox = dd;
oy = -dd;
alpha = -pi/4;

dx = xB - ox;                               % 다리 원점 기준 x 거리를 계산한다.
dy = yB - oy;                               % 다리 원점 기준 y 거리를 계산한다.

xL =  dx*cos(alpha) + dy*sin(alpha);         % 다리 x 위치를 계산한다.
yL = -dx*sin(alpha) + dy*cos(alpha);         % 다리 y 위치를 계산한다.
zL =  zB;                                    % 다리 z 위치를 전달한다.
end

== matlab function plant/MATLAB Function14 ==
  data: xB input; xL output; yB input; zB input; yL output; zL output
function [xL, yL, zL] = bodyToLeg(xB, yB, zB)
% Body 좌표의 발 목표를 다리 좌표로 변환한다.

% 몸체의 원점에서 링크1 까지 거리 (m)
d = 0.1845;
dd = d / sqrt(2);

ox = 0;
oy = -d;
alpha = -pi/2;

dx = xB - ox;                               % 다리 원점 기준 x 거리를 계산한다.
dy = yB - oy;                               % 다리 원점 기준 y 거리를 계산한다.

xL =  dx*cos(alpha) + dy*sin(alpha);         % 다리 x 위치를 계산한다.
yL = -dx*sin(alpha) + dy*cos(alpha);         % 다리 y 위치를 계산한다.
zL =  zB;                                    % 다리 z 위치를 전달한다.
end

== matlab function plant/MATLAB Function15 ==
  data: xB input; xL output; yB input; zB input; yL output; zL output
function [xL, yL, zL] = bodyToLeg(xB, yB, zB)
% Body 좌표의 발 목표를 다리 좌표로 변환한다.

% 몸체의 원점에서 링크1 까지 거리 (m)
d = 0.1845;
dd = d / sqrt(2);

ox = -dd;
oy = -dd;
alpha = -3*pi/4;

dx = xB - ox;                               % 다리 원점 기준 x 거리를 계산한다.
dy = yB - oy;                               % 다리 원점 기준 y 거리를 계산한다.

xL =  dx*cos(alpha) + dy*sin(alpha);         % 다리 x 위치를 계산한다.
yL = -dx*sin(alpha) + dy*cos(alpha);         % 다리 y 위치를 계산한다.
zL =  zB;                                    % 다리 z 위치를 전달한다.
end

== matlab function plant/MATLAB Function16 ==
  data: xB input; xL output; yB input; zB input; yL output; zL output
function [xL, yL, zL] = bodyToLeg(xB, yB, zB)
% Body 좌표의 발 목표를 다리 좌표로 변환한다.

% 몸체의 원점에서 링크1 까지 거리 (m)
d = 0.1845;
dd = d / sqrt(2);

ox = dd;
oy = dd;
alpha = pi/4;

dx = xB - ox;                               % 다리 원점 기준 x 거리를 계산한다.
dy = yB - oy;                               % 다리 원점 기준 y 거리를 계산한다.

xL =  dx*cos(alpha) + dy*sin(alpha);         % 다리 x 위치를 계산한다.
yL = -dx*sin(alpha) + dy*cos(alpha);         % 다리 y 위치를 계산한다.
zL =  zB;                                    % 다리 z 위치를 전달한다.
end

== matlab function plant/MATLAB Function17 ==
  data: xB input; xL output; yB input; zB input; yL output; zL output
function [xL, yL, zL] = bodyToLeg(xB, yB, zB)
% Body 좌표의 발 목표를 다리 좌표로 변환한다.

% 몸체의 원점에서 링크1 까지 거리 (m)
d = 0.1845;
dd = d / sqrt(2);

ox = 0;
oy = d;
alpha = pi/2;

dx = xB - ox;                               % 다리 원점 기준 x 거리를 계산한다.
dy = yB - oy;                               % 다리 원점 기준 y 거리를 계산한다.

xL =  dx*cos(alpha) + dy*sin(alpha);         % 다리 x 위치를 계산한다.
yL = -dx*sin(alpha) + dy*cos(alpha);         % 다리 y 위치를 계산한다.
zL =  zB;                                    % 다리 z 위치를 전달한다.
end

== matlab function plant/MATLAB Function18 ==
  data: xB input; xL output; yB input; zB input; yL output; zL output
function [xL, yL, zL] = bodyToLeg(xB, yB, zB)
% Body 좌표의 발 목표를 다리 좌표로 변환한다.

% 몸체의 원점에서 링크1 까지 거리 (m)
d = 0.1845;
dd = d / sqrt(2);

ox = -dd;
oy = dd;
alpha = 3*pi/4;

dx = xB - ox;                               % 다리 원점 기준 x 거리를 계산한다.
dy = yB - oy;                               % 다리 원점 기준 y 거리를 계산한다.

xL =  dx*cos(alpha) + dy*sin(alpha);         % 다리 x 위치를 계산한다.
yL = -dx*sin(alpha) + dy*cos(alpha);         % 다리 y 위치를 계산한다.
zL =  zB;                                    % 다리 z 위치를 전달한다.
end

== matlab function plant/MATLAB Function19 ==
  data: x input; q1 output; y input; z input; q2 output; q3 output
function [q1, q2, q3] = legIK(x, y, z)
% 발 목표 위치로 관절 목표각을 계산한다.

L1 = 0.074;   % 링크1 에서 링크1 까지 거리 (m)
L2 = 0.121;   % 링크2 에서 링크3 까지 거리 (m)
L3 = 0.230;   % 링크3 에서 발 끝 까지 거리 (m)

r_xy = sqrt(x*x + y*y);                      % 수평 거리를 계산한다.
u = r_xy - L1;                               % 2번 관절 기준 거리를 계산한다.

c3 = (u*u + z*z - L2*L2 - L3*L3) ...
   / (2*L2*L3);                              % 3번 관절 코사인을 계산한다.

assert(abs(c3) <= 1.000001);                  % IK 도달 가능 영역을 확인한다.

c3 = min(max(c3, -1), 1);                    % 수치 오차를 제한한다.
s3 = sqrt(max(0, 1 - c3*c3));                % 양의 무릎 방향을 선택한다.

q1 = atan2(y, x);                            % 1번 관절각을 계산한다.
q3 = atan2(s3, c3);                          % 3번 관절각을 계산한다.
q2 = atan2(-z, u) ...
   - atan2(L3*s3, L2 + L3*c3);               % 2번 관절각을 계산한다.
end

== matlab function plant/MATLAB Function20 ==
  data: x input; q1 output; y input; z input; q2 output; q3 output
function [q1, q2, q3] = legIK(x, y, z)
% 발 목표 위치로 관절 목표각을 계산한다.

L1 = 0.074;   % 링크1 에서 링크1 까지 거리 (m)
L2 = 0.121;   % 링크2 에서 링크3 까지 거리 (m)
L3 = 0.230;   % 링크3 에서 발 끝 까지 거리 (m)

r_xy = sqrt(x*x + y*y);                      % 수평 거리를 계산한다.
u = r_xy - L1;                               % 2번 관절 기준 거리를 계산한다.

c3 = (u*u + z*z - L2*L2 - L3*L3) ...
   / (2*L2*L3);                              % 3번 관절 코사인을 계산한다.

assert(abs(c3) <= 1.000001);                  % IK 도달 가능 영역을 확인한다.

c3 = min(max(c3, -1), 1);                    % 수치 오차를 제한한다.
s3 = sqrt(max(0, 1 - c3*c3));                % 양의 무릎 방향을 선택한다.

q1 = atan2(y, x);                            % 1번 관절각을 계산한다.
q3 = atan2(s3, c3);                          % 3번 관절각을 계산한다.
q2 = atan2(-z, u) ...
   - atan2(L3*s3, L2 + L3*c3);               % 2번 관절각을 계산한다.
end

== matlab function plant/MATLAB Function21 ==
  data: x input; q1 output; y input; z input; q2 output; q3 output
function [q1, q2, q3] = legIK(x, y, z)
% 발 목표 위치로 관절 목표각을 계산한다.

L1 = 0.074;   % 링크1 에서 링크1 까지 거리 (m)
L2 = 0.121;   % 링크2 에서 링크3 까지 거리 (m)
L3 = 0.230;   % 링크3 에서 발 끝 까지 거리 (m)

r_xy = sqrt(x*x + y*y);                      % 수평 거리를 계산한다.
u = r_xy - L1;                               % 2번 관절 기준 거리를 계산한다.

c3 = (u*u + z*z - L2*L2 - L3*L3) ...
   / (2*L2*L3);                              % 3번 관절 코사인을 계산한다.

assert(abs(c3) <= 1.000001);                  % IK 도달 가능 영역을 확인한다.

c3 = min(max(c3, -1), 1);                    % 수치 오차를 제한한다.
s3 = sqrt(max(0, 1 - c3*c3));                % 양의 무릎 방향을 선택한다.

q1 = atan2(y, x);                            % 1번 관절각을 계산한다.
q3 = atan2(s3, c3);                          % 3번 관절각을 계산한다.
q2 = atan2(-z, u) ...
   - atan2(L3*s3, L2 + L3*c3);               % 2번 관절각을 계산한다.
end

== matlab function plant/MATLAB Function22 ==
  data: x input; q1 output; y input; z input; q2 output; q3 output
function [q1, q2, q3] = legIK(x, y, z)
% 발 목표 위치로 관절 목표각을 계산한다.

L1 = 0.074;   % 링크1 에서 링크1 까지 거리 (m)
L2 = 0.121;   % 링크2 에서 링크3 까지 거리 (m)
L3 = 0.230;   % 링크3 에서 발 끝 까지 거리 (m)

r_xy = sqrt(x*x + y*y);                      % 수평 거리를 계산한다.
u = r_xy - L1;                               % 2번 관절 기준 거리를 계산한다.

c3 = (u*u + z*z - L2*L2 - L3*L3) ...
   / (2*L2*L3);                              % 3번 관절 코사인을 계산한다.

assert(abs(c3) <= 1.000001);                  % IK 도달 가능 영역을 확인한다.

c3 = min(max(c3, -1), 1);                    % 수치 오차를 제한한다.
s3 = sqrt(max(0, 1 - c3*c3));                % 양의 무릎 방향을 선택한다.

q1 = atan2(y, x);                            % 1번 관절각을 계산한다.
q3 = atan2(s3, c3);                          % 3번 관절각을 계산한다.
q2 = atan2(-z, u) ...
   - atan2(L3*s3, L2 + L3*c3);               % 2번 관절각을 계산한다.
end

== matlab function plant/MATLAB Function23 ==
  data: x input; q1 output; y input; z input; q2 output; q3 output
function [q1, q2, q3] = legIK(x, y, z)
% 발 목표 위치로 관절 목표각을 계산한다.

L1 = 0.074;   % 링크1 에서 링크1 까지 거리 (m)
L2 = 0.121;   % 링크2 에서 링크3 까지 거리 (m)
L3 = 0.230;   % 링크3 에서 발 끝 까지 거리 (m)

r_xy = sqrt(x*x + y*y);                      % 수평 거리를 계산한다.
u = r_xy - L1;                               % 2번 관절 기준 거리를 계산한다.

c3 = (u*u + z*z - L2*L2 - L3*L3) ...
   / (2*L2*L3);                              % 3번 관절 코사인을 계산한다.

assert(abs(c3) <= 1.000001);                  % IK 도달 가능 영역을 확인한다.

c3 = min(max(c3, -1), 1);                    % 수치 오차를 제한한다.
s3 = sqrt(max(0, 1 - c3*c3));                % 양의 무릎 방향을 선택한다.

q1 = atan2(y, x);                            % 1번 관절각을 계산한다.
q3 = atan2(s3, c3);                          % 3번 관절각을 계산한다.
q2 = atan2(-z, u) ...
   - atan2(L3*s3, L2 + L3*c3);               % 2번 관절각을 계산한다.
end

== matlab function plant/MATLAB Function24 ==
  data: x input; q1 output; y input; z input; q2 output; q3 output
function [q1, q2, q3] = legIK(x, y, z)
% 발 목표 위치로 관절 목표각을 계산한다.

L1 = 0.074;   % 링크1 에서 링크1 까지 거리 (m)
L2 = 0.121;   % 링크2 에서 링크3 까지 거리 (m)
L3 = 0.230;   % 링크3 에서 발 끝 까지 거리 (m)

r_xy = sqrt(x*x + y*y);                      % 수평 거리를 계산한다.
u = r_xy - L1;                               % 2번 관절 기준 거리를 계산한다.

c3 = (u*u + z*z - L2*L2 - L3*L3) ...
   / (2*L2*L3);                              % 3번 관절 코사인을 계산한다.

assert(abs(c3) <= 1.000001);                  % IK 도달 가능 영역을 확인한다.

c3 = min(max(c3, -1), 1);                    % 수치 오차를 제한한다.
s3 = sqrt(max(0, 1 - c3*c3));                % 양의 무릎 방향을 선택한다.

q1 = atan2(y, x);                            % 1번 관절각을 계산한다.
q3 = atan2(s3, c3);                          % 3번 관절각을 계산한다.
q2 = atan2(-z, u) ...
   - atan2(L3*s3, L2 + L3*c3);               % 2번 관절각을 계산한다.
end

== matlab function plant/MATLAB Function25 ==
  data: t input; vx output; vy output; vz output; wx output; wy output; wz output
function [vx, vy, vz, wx, wy, wz] = TestBodyTwist(t)

vx = 0;
vy = 0;   % 사실상 0
vz = 0;   % 사실상 0

wx = 0;   % 0인지 아닌지 모르겠음
wy = 0;   % 0인지 아닌지 모르겠음
wz = 0;

% Tripod 보행 시작과 동시에 전진 명령을 적용한다.
if t >= 1.0
    vx = 0.14; % 최대 속도 2km/h(0.28m/s)
end

end

== matlab function plant/Plant/MATLAB Function ==
  data: t input; Contact1 output; Contact2 output; Contact3 output; Contact4 output; Contact5 output; Contact6 output
% Tripod Gait의 기본 접촉 신호를 반복 생성한다.
function [Contact1, Contact2, Contact3, ...
          Contact4, Contact5, Contact6] = TestContact(t)

Gait_Start_Time = 1.0;    % 보행 시작 시간을 정의한다.
Phase_Time      = 0.60;   % 한 Phase의 시간을 정의한다.
Landing_Time    = 0.50;   % Swing 다리의 정상 착지 시간을 정의한다.

% 보행 시작 전에는 모든 발을 접촉 상태로 둔다.
Contact1 = 1;
Contact2 = 1;
Contact3 = 1;
Contact4 = 1;
Contact5 = 1;
Contact6 = 1;

if t < Gait_Start_Time
    return;
end

% 현재 Phase와 Phase 내부 시간을 계산한다.
elapsed_time = t - Gait_Start_Time;

phase_count = floor(elapsed_time / Phase_Time);
phase_time  = elapsed_time - phase_count * Phase_Time;

% 짝수 Phase : 1, 3, 5번 다리 Swing
if mod(phase_count, 2) == 0

    Contact1 = double(phase_time >= Landing_Time);
    Contact3 = double(phase_time >= Landing_Time);
    Contact5 = double(phase_time >= Landing_Time);

% 홀수 Phase : 2, 4, 6번 다리 Swing
else

    Contact2 = double(phase_time >= Landing_Time);
    Contact4 = double(phase_time >= Landing_Time);
    Contact6 = double(phase_time >= Landing_Time);

end

end

== matlab function plant/MATLAB Function27 ==
  data: t input; Leg1_State output; Leg1_Progress output; Leg2_State output; Leg2_Progress output; Leg3_State output; Leg3_Progress output; Leg4_State output; Leg4_Progress output; Leg5_State output; Leg5_Progress output; Leg6_State output; Leg6_Progress output; Startup_Phase output; leg_1_press input; leg_2_press input; leg_3_press input; leg_4_press input; leg_5_press input; leg_6_press input
% Contact를 반영하여 6개 다리의 보행 상태와 진행률을 계산한다.
function [Leg1_State, Leg1_Progress, ...
          Leg2_State, Leg2_Progress, ...
          Leg3_State, Leg3_Progress, ...
          Leg4_State, Leg4_Progress, ...
          Leg5_State, Leg5_Progress, ...
          Leg6_State, Leg6_Progress, ...
          Startup_Phase] = TripodGaitManager( ...
          t, leg_1_press, leg_2_press, leg_3_press, leg_4_press, leg_5_press, leg_6_press)

STANCE       = 0;  % Stance 상태 번호를 정의한다.
SWING        = 1;  % Swing 상태 번호를 정의한다.
LATE_LANDING = 2;  % Late Landing 상태 번호를 정의한다.

Gait_Start_Time    = 1.0;  % 보행 시작 시간을 정의한다.
Phase_Time         = 0.5;  % 한 Tripod Phase 시간을 정의한다.
Early_Min_Progress = 0.5;  % Swing 하강 구간부터 접촉을 인정한다.

persistent Initialized Phase_Index Phase_Start_Time
persistent Airborne_Seen Landed

if isempty(Initialized)
    Initialized      = false;
    Phase_Index      = 0;
    Phase_Start_Time = Gait_Start_Time;
    Airborne_Seen    = false(1, 6);
    Landed           = false(1, 6);
end

% 보행 시작 전에는 상태 메모리를 초기화한다.
if t < Gait_Start_Time
    Initialized      = false;
    Phase_Index      = 0;
    Phase_Start_Time = Gait_Start_Time;
    Airborne_Seen(:) = false;
    Landed(:)        = false;

    Leg1_State = STANCE;
    Leg2_State = STANCE;
    Leg3_State = STANCE;
    Leg4_State = STANCE;
    Leg5_State = STANCE;
    Leg6_State = STANCE;

    Leg1_Progress = 0;
    Leg2_Progress = 0;
    Leg3_Progress = 0;
    Leg4_Progress = 0;
    Leg5_Progress = 0;
    Leg6_Progress = 0;

    Startup_Phase = 1;
    return;
end

% 보행 시작 시 첫 Phase 기준 시간을 설정한다.
if ~Initialized
    Initialized      = true;
    Phase_Index      = 0;
    Phase_Start_Time = Gait_Start_Time;
    Airborne_Seen(:) = false;
    Landed(:)        = false;
end

contacts = [leg_1_press ~= 0, leg_2_press ~= 0, leg_3_press ~= 0, ...
            leg_4_press ~= 0, leg_5_press ~= 0, leg_6_press ~= 0];

% 현재 Phase 진행률을 계산한다.
phase_progress = (t - Phase_Start_Time)/Phase_Time;

if phase_progress < 0
    phase_progress = 0;
elseif phase_progress > 1
    phase_progress = 1;
end

% 현재 Swing 그룹을 선택한다.
if mod(Phase_Index, 2) == 0
    swing_mask = [true, false, true, false, true, false];
else
    swing_mask = [false, true, false, true, false, true];
end

% 미접촉을 확인한 이후의 재접촉만 착륙으로 인정한다.
for i = 1:6
    if swing_mask(i)
        if ~contacts(i)
            Airborne_Seen(i) = true;
        end

        if Airborne_Seen(i) && contacts(i) && ...
                phase_progress >= Early_Min_Progress
            Landed(i) = true;
        end
    end
end

% 현재 Swing 그룹의 착륙 완료 여부를 계산한다.
all_swing_landed = true;

for i = 1:6
    if swing_mask(i) && ~Landed(i)
        all_swing_landed = false;
    end
end

% 정상 시간이 끝나고 모두 착륙하면 다음 Phase로 전환한다.
if phase_progress >= 1 && all_swing_landed
    Phase_Index      = Phase_Index + 1;
    Phase_Start_Time = t;
    Airborne_Seen(:) = false;
    Landed(:)        = false;
    phase_progress   = 0;

    if mod(Phase_Index, 2) == 0
        swing_mask = [true, false, true, false, true, false];
    else
        swing_mask = [false, true, false, true, false, true];
    end
end

% 다리별 최종 상태를 결정한다.
states = zeros(1, 6);

for i = 1:6
    if ~swing_mask(i)
        states(i) = STANCE;

    elseif Landed(i)
        states(i) = STANCE;

    elseif phase_progress >= 1
        states(i) = LATE_LANDING;

    else
        states(i) = SWING;
    end
end

Leg1_State = states(1);
Leg2_State = states(2);
Leg3_State = states(3);
Leg4_State = states(4);
Leg5_State = states(5);
Leg6_State = states(6);

Leg1_Progress = phase_progress;
Leg2_Progress = phase_progress;
Leg3_Progress = phase_progress;
Leg4_Progress = phase_progress;
Leg5_Progress = phase_progress;
Leg6_Progress = phase_progress;

Startup_Phase = double(Phase_Index == 0);

end
